simulink model "L1_B"  (R2020a)
settings: Solver=VariableStepAuto  StartTime=0.0  StopTime=10.0  RelTol=1e-3
settings Model: Creator=fbi  LastModifiedBy=fbi

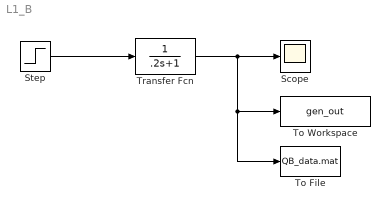
== system L1_B ==
  Scope : Scope
  Step : Step  Time=0  SampleTime=0
  To File : ToFile  Filename=QB_data.mat  MatrixName=gen_out  SaveFormat=Timeseries
  To Workspace : ToWorkspace  VariableName=gen_out  SampleTime=-1
  Transfer Fcn : TransferFcn  Denominator=[.2 1]
  wires:
  Step/1 -> Transfer Fcn/1
  Transfer Fcn/1 -> To File/1, To Workspace/1, Scope/1
